simulink model "ex1_2"  (R2016a)
settings: Solver=VariableStepAuto  StartTime=0.0  StopTime=10.0  RelTol=1e-3
libraries: simulink x3
settings Model: Creator=Utilizator  LastModifiedBy=Utilizator

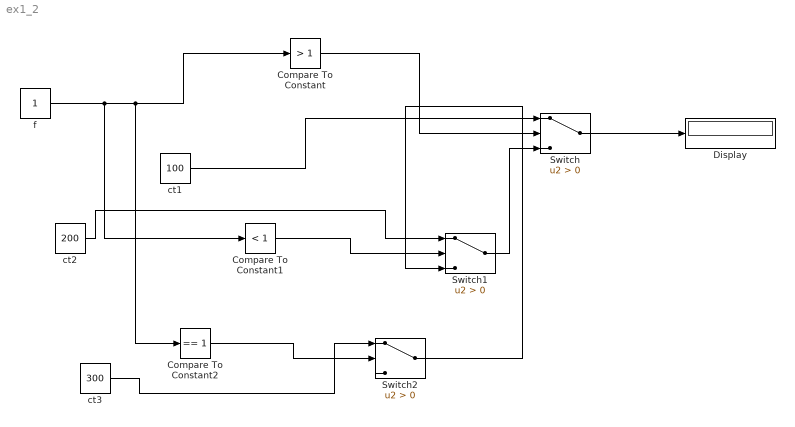
== system ex1_2 ==
  Compare To Constant : simulink/Logic and Bit Operations/Compare To Constant  relop=>  const=1  OutDataTypeStr=boolean
  Compare To Constant1 : simulink/Logic and Bit Operations/Compare To Constant  relop=<  const=1  OutDataTypeStr=boolean
  Compare To Constant2 : simulink/Logic and Bit Operations/Compare To Constant  relop===  const=1  OutDataTypeStr=boolean
  Display : Display
  Switch : Switch  Criteria=u2 > Threshold
  Switch1 : Switch  Criteria=u2 > Threshold
  Switch2 : Switch  Criteria=u2 > Threshold
  ct1 : Constant  Value=100
  ct2 : Constant  Value=200
  ct3 : Constant  Value=300
  f : Constant
  wires:
  ct1/1 -> Switch/1
  f/1 -> Compare To Constant1/1, Compare To Constant2/1, Compare To Constant/1
  Compare To Constant/1 -> Switch/2
  Switch1/1 -> Switch/3
  Compare To Constant1/1 -> Switch1/2
  ct2/1 -> Switch1/1
  Switch/1 -> Display/1
  Compare To Constant2/1 -> Switch2/2
  ct3/1 -> Switch2/1
  Switch2/1 -> Switch1/3
